simulink model "model"  (R2023b)
settings: Solver=VariableStepAuto  StartTime=0.0  StopTime=1000  RelTol=1e-3
values from neighbouring files (symbols this model uses):
  a = ones(size(R))    [static_characteristic_u_y.m]
  c = [10 25 40 55 70]    [static_characteristic_u_y.m]
  F_10 = 90    [PID_controller_fuzzy.m]
  h_20 = 36    [PID_controller_fuzzy.m]
  tau = 2    [GPC_analitic.m]    (also in GPC_analitic_Bezout.m)
undefined symbols (not defined in the file or in its folder): alpha_1, alpha_2, F_D0, G_s, h_10
libraries: fuzblock x1
settings Model: Creator=HP  LastModifiedBy=HP

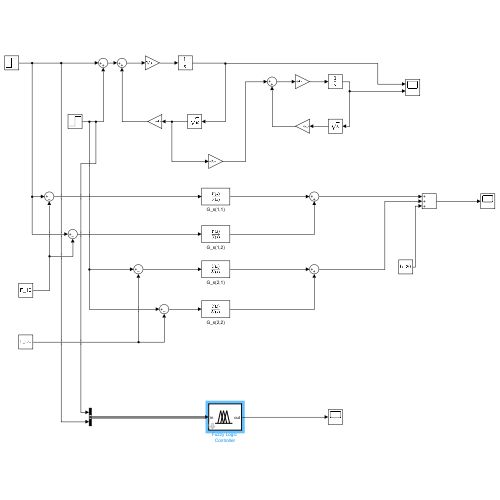
[thumbnail: Simulink's stored preview of the top-level diagram]
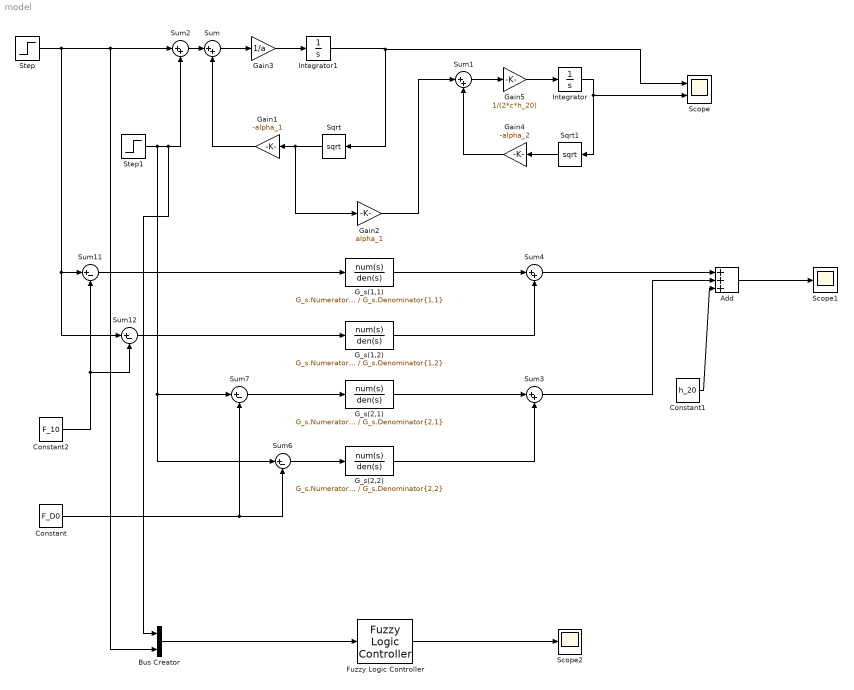
== system model ==
  Add : Sum  Inputs=+++
  Bus Creator : BusCreator  Inputs=2
  Constant : Constant  Value=F_D0
  Constant1 : Constant  Value=h_20
  Constant2 : Constant  Value=F_10
  Fuzzy Logic Controller : fuzblock/Fuzzy Logic  Controller  FIS=FIS  OutputSampleNumber=101  DataType=double  FuzzifiedInputs=off  RuleFiringStrengths=off  RuleOutputs=off  AggregatedOutputs=off  SimulateUsing=Interpreted execution  OutOfRangeInputValueMessage=warning  NoRuleFiredMessage=warning  EmptyOutputFuzzySetMessage=warning
  G_s(1,1) : TransferFcn  Numerator=G_s.Numerator{1,1}  Denominator=G_s.Denominator{1,1}
  G_s(1,2) : TransferFcn  Numerator=G_s.Numerator{1,2}  Denominator=G_s.Denominator{1,2}
  G_s(2,1) : TransferFcn  Numerator=G_s.Numerator{2,1}  Denominator=G_s.Denominator{2,1}
  G_s(2,2) : TransferFcn  Numerator=G_s.Numerator{2,2}  Denominator=G_s.Denominator{2,2}
  Gain1 : Gain  Gain=-alpha_1
  Gain2 : Gain  Gain=alpha_1
  Gain3 : Gain  Gain=1/a
  Gain4 : Gain  Gain=-alpha_2
  Gain5 : Gain  Gain=1/(2*c*h_20)
  Integrator : Integrator  InitialCondition=h_20
  Integrator1 : Integrator  InitialCondition=h_10
  Scope : Scope  NumInputPorts=2
  Scope1 : Scope
  Scope2 : Scope
  Sqrt : Sqrt
  Sqrt1 : Sqrt
  Step : Step  Time=tau  Before=F_10  After=F_10 + 10  SampleTime=0
  Step1 : Step  Time=0  After=F_D0  SampleTime=0
  Sum{,1..4} (5 alike) : Sum  Inputs=|++
  Sum{6..7,11..12} (4 alike) : Sum  Inputs=|+-
  wires:
  Sum/1 -> Gain3/1
  Integrator1/1 -> Sqrt/1, Scope/1
  Sqrt/1 -> Gain1/1, Gain2/1
  Gain1/1 -> Sum/2
  Gain2/1 -> Sum1/1
  Sum1/1 -> Gain5/1
  Integrator/1 -> Sqrt1/1, Scope/2
  Sqrt1/1 -> Gain4/1
  Gain4/1 -> Sum1/2
  Gain3/1 -> Integrator1/1
  Gain5/1 -> Integrator/1
  Step1/1 -> Sum6/1, Sum7/1, Bus Creator/1, Sum2/2
  Step/1 -> Bus Creator/2, Sum2/1, Sum12/1, Sum11/1
  Sum2/1 -> Sum/1
  G_s(1,1)/1 -> Sum4/1
  G_s(1,2)/1 -> Sum4/2
  G_s(2,1)/1 -> Sum3/1
  G_s(2,2)/1 -> Sum3/2
  Sum4/1 -> Add/1
  Sum3/1 -> Add/2
  Add/1 -> Scope1/1
  Constant/1 -> Sum6/2, Sum7/2
  Sum7/1 -> G_s(2,1)/1
  Sum6/1 -> G_s(2,2)/1
  Sum11/1 -> G_s(1,1)/1
  Sum12/1 -> G_s(1,2)/1
  Constant2/1 -> Sum12/2, Sum11/2
  Constant1/1 -> Add/3
  Bus Creator/1 -> Fuzzy Logic Controller/1
  Fuzzy Logic Controller/1 -> Scope2/1
